simulink model "MSFS_SITL_Roll_Controller"  (R2022a)
settings: Solver=FixedStepDiscrete  StartTime=0.0  StopTime=inf  FixedStep=0.03  RelTol=1e-3
libraries: SimConnectToolbox x4, simulink_extras x3, slpidlib x1
settings Model: Creator=Andreas  LastModifiedBy=Alireza
settings SolverCC: AlgebraicLoopSolver=TrustRegion
settings DebuggingCC: InheritedTsInSrcMsg=none  UnconnectedInputMsg=warning  UnconnectedOutputMsg=warning  UnconnectedLineMsg=warning  SFMachineParentedDataDiag=warning
settings RTWCC: DLArmComputeVersion=19.05

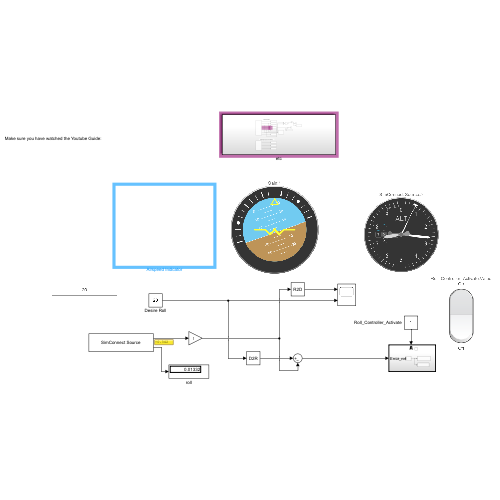
[thumbnail: Simulink's stored preview of the top-level diagram]
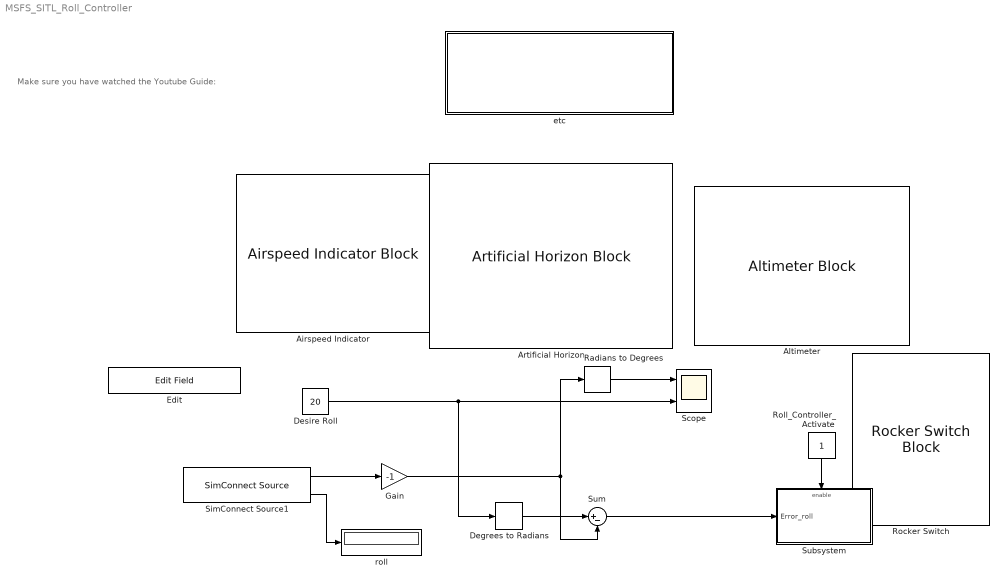
== system MSFS_SITL_Roll_Controller ==
  note: Make sure you have watched the Youtube Guide:
  Airspeed Indicator : AirspeedIndicatorBlock
  Altimeter : AltimeterBlock
  Artificial Horizon : ArtificialHorizonBlock
  Degrees to Radians : simulink_extras/Transformations/Degrees to Radians
  Desire Roll : Constant  Value=20
  Edit : EditField  LabelPosition=Hide  ShowInitialText=on  Alignment=Center
  Gain : Gain  Gain=-1
  Radians to Degrees : simulink_extras/Transformations/Radians to Degrees
  Rocker Switch : RockerSwitchBlock
      settings: Values={{'Off', 'On'}, [0 1]}
  Roll_Controller_Activate : Constant
  Scope : Scope  NumInputPorts=2
  SimConnect Source1 : SimConnectToolbox/SimConnect Source  configurationIndex=0  connectionName=SimConnectSource  variables=|
      | PLANE BANK DEGREES, RADIANS;
      | AILERON POSITION, POSITION;
      settings: SourceProductName=SimConnect Toolbox
  Subsystem : Subsystem
  Sum : Sum  Inputs=|+-
  etc : Subsystem
  roll : Display
  wires:
  Radians to Degrees/1 -> Scope/1
  SimConnect Source1/2 -> roll/1
  SimConnect Source1/1 -> Gain/1
  Degrees to Radians/1 -> Sum/1
  Desire Roll/1 -> Degrees to Radians/1, Scope/2
  Sum/1 -> Subsystem/1(Error_roll)
  Roll_Controller_Activate/1 -> Subsystem/Enable
  Gain/1 -> Radians to Degrees/1, Sum/2

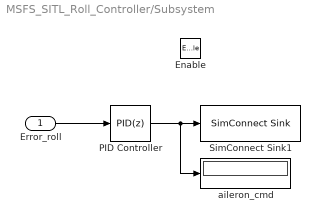
== system MSFS_SITL_Roll_Controller/Subsystem ==
  Error_roll : Inport
  Enable : EnablePort
  PID Controller : slpidlib/PID Controller  Controller=PID  Form=Parallel  TimeDomain=Discrete-time  UseExternalTs=off  SampleTime=-1  IntegratorMethod=Forward Euler  FilterMethod=Forward Euler  ControllerParametersSource=internal  P=1  I=1  UseKiTs=off  D=0  N=100  UseFilter=on  TunerSelectOption=Transfer Function Based (PID Tuner App)  InitialConditionSource=internal  InitialConditionForIntegrator=0  InitialConditionForFilter=0  DifferentiatorICPrevScaledInput=0  ExternalReset=none  TrackingMode=off  Kt=1  LimitOutput=on  SatLimitsSource=internal  UpperSaturationLimit=1  LowerSaturationLimit=-1  LinearizeAsGain=on  AntiWindupMode=none  Kb=1  POutMin=[]  POutMax=[]  IOutMin=[]  IOutMax=[]  DOutMin=[]  DOutMax=[]  NOutMin=[]  NOutMax=[]  SumOutMin=[]  SumOutMax=[]  SaturationOutMin=[]  SaturationOutMax=[]  PParamMin=[]  PParamMax=[]  IParamMin=[]  IParamMax=[]  DParamMin=[]  DParamMax=[]  NParamMin=[]  NParamMax=[]  KbParamMin=[]  KbParamMax=[]  KtParamMin=[]  KtParamMax=[]  KbOutMin=[]  KbOutMax=[]  KtOutMin=[]  KtOutMax=[]  IntegratorOutMin=[]  IntegratorOutMax=[]  FilterOutMin=[]  FilterOutMax=[]  SumI1OutMin=[]  SumI1OutMax=[]  SumI2OutMin=[]  SumI2OutMax=[]  SumI3OutMin=[]  SumI3OutMax=[]  SumI4OutMin=[]  SumI4OutMax=[]  SumDOutMin=[]  SumDOutMax=[]  DifferentiatorOutMin=[]  DifferentiatorOutMax=[]  FilterDiffOutCoefMin=[]  FilterDiffOutCoefMax=[]  ReciprocalOutMin=[]  ReciprocalOutMax=[]  SumDenOutMin=[]  SumDenOutMax=[]  SumNumOutMin=[]  SumNumOutMax=[]  DivideOutMin=[]  DivideOutMax=[]  UdiffTsProdOutMin=[]  UdiffTsProdOutMax=[]  NTsProdOutMin=[]  NTsProdOutMax=[]  UintegralTsProdOutMin=[]  UintegralTsProdOutMax=[]  UngainTsProdOutMin=[]  UngainTsProdOutMax=[]  IntegratorContinuousStateAttributes=''  IntegratorStateMustResolveToSignalObject=off  IntegratorRTWStateStorageClass=Auto  FilterContinuousStateAttributes=''  FilterStateMustResolveToSignalObject=off  FilterRTWStateStorageClass=Auto  ParallelPVariant=InternalParameters  IdealPVariant=Disabled  IVariant=InternalParameters  DVariant=InternalParameters  IntegratorVariant=Discrete  SatVariant=Enabled  AWVariant=Passthrough  PCopyVariant=Disabled  TRVariant=Disabled  FdbkBlocksVariant=Forward  IdealPFdbkVariant=Disabled  SatFdbkVariant=Disabled  DerivativeFilterVariant=ForwardEulerFilter  NVariant=InternalParameters  NCopyVariant=Disabled  FilterICVariant=InternalICsFilter  IntegratorICVariant=InternalICs  ExternalResetVariant=Disabled  TRSumVariant=Passthrough  SumFdbkVariant=Disabled  SumVariant=Sum_PID  TsampFilterVariant=InternalTs  TsampNgainVariant=Passthrough  TsampIntegralVariant=Passthrough  ExternalSaturationOutDataTypeStr=Inherit: Same as second input  aMode=0
  SimConnect Sink1 : SimConnectToolbox/SimConnect Sink  configurationIndex=0  connectionName=SimConnectSink  variables=AILERON POSITION, POSITION;
      settings: SourceProductName=SimConnect Toolbox
  aileron_cmd : Display
  wires:
  Error_roll/1 -> PID Controller/1
  PID Controller/1 -> SimConnect Sink1/1, aileron_cmd/1

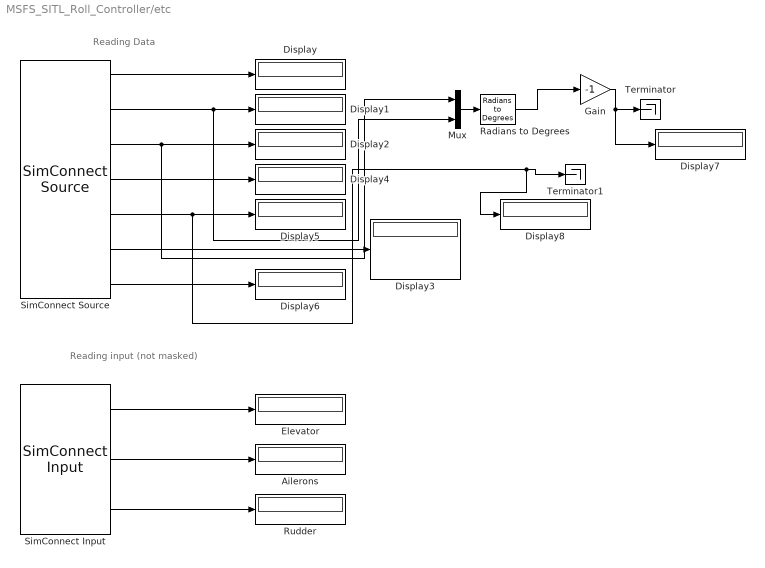
== system MSFS_SITL_Roll_Controller/etc ==
  note: Reading input (not masked)
  note: Reading Data
  Ailerons : Display
  Display{,1..8} (9 alike) : Display
  Elevator : Display
  Gain : Gain  Gain=-1
  Mux : Mux  Inputs=2
  Radians to Degrees : simulink_extras/Transformations/Radians to Degrees
  Rudder : Display
  SimConnect Input : SimConnectToolbox/SimConnect Input  configurationIndex=0  connectionName=SimConnectInput  variables=|
      | AXIS_ELEVATOR_SET, FALSE;
      | AXIS_AILERONS_SET, FALSE;
      | AXIS_RUDDER_SET, FALSE;
      settings: SourceProductName=SimConnect Toolbox
      mask Display:
      | % This is a new mask on top of the base mask.
      | % Use "View base mask" link below to see the base mask.
      | port_label('output', 1, '\delta_\eta', 'texmode', 'on')
      | port_label('output', 2, '\delta_\xi', 'texmode', 'on')
      | port_label('output', 3, '\delta_\zeta', 'texmode', 'on')
  SimConnect Source : SimConnectToolbox/SimConnect Source  configurationIndex=0  connectionName=SimConnectSource  variables=|
      | G FORCE, GFORCE;
      | PLANE PITCH DEGREES, RADIANS;
      | PLANE BANK DEGREES, RADIANS;
      | AIRSPEED INDICATED, KNOTS;
      | PLANE ALTITUDE, FEET;
      | STRUCT WORLD ROTATION VELOCITY, STRUCT;
      | LIGHT STROBE ON, BOOL;
      settings: SourceProductName=SimConnect Toolbox
      mask Display:
      | % This is a new mask on top of the base mask.
      | % Use "View base mask" link below to see the base mask.
      | port_label('output', 1, 'g', 'texmode', 'on')
      | port_label('output', 2, '\Theta (rad)', 'texmode', 'on')
      | port_label('output', 3, '\Phi (rad)', 'texmode', 'on')
      | port_label('output', 4, 'IAS (kts)', 'texmode', 'on')
      | port_label('output', 5, 'Alt (ft)', 'texmode', 'on')
      | port_label('output', 6, 'World R-Velocity', 'texmode', 'on')
      | port_label('output', 7, 'Strobe-Light On', 'texmode', 'on')
  Terminator : Terminator
  Terminator1 : Terminator
  wires:
  SimConnect Source/3 -> Mux/1, Display2/1
  SimConnect Source/6 -> Display3/1
  SimConnect Source/1 -> Display/1
  Radians to Degrees/1 -> Gain/1
  SimConnect Input/2 -> Ailerons/1
  SimConnect Source/7 -> Display6/1
  SimConnect Source/5 -> Display8/1, Terminator1/1, Display5/1
  SimConnect Source/2 -> Mux/2, Display1/1
  SimConnect Input/3 -> Rudder/1
  Mux/1 -> Radians to Degrees/1
  SimConnect Input/1 -> Elevator/1
  SimConnect Source/4 -> Display4/1
  Gain/1 -> Display7/1, Terminator/1
